simulink model "mass_spring_damper"  (R2026a)
settings: Solver=VariableStepAuto  StopTime=10

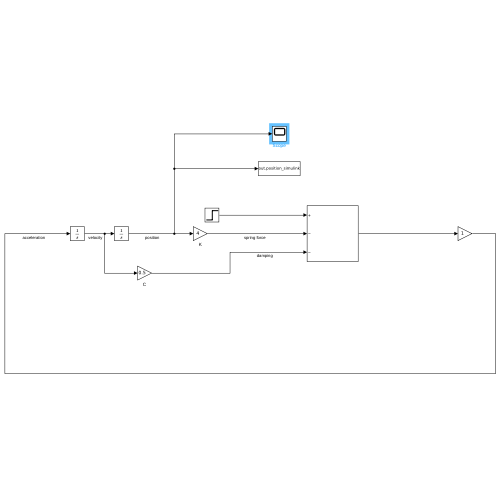
[thumbnail: Simulink's stored preview of the top-level diagram]
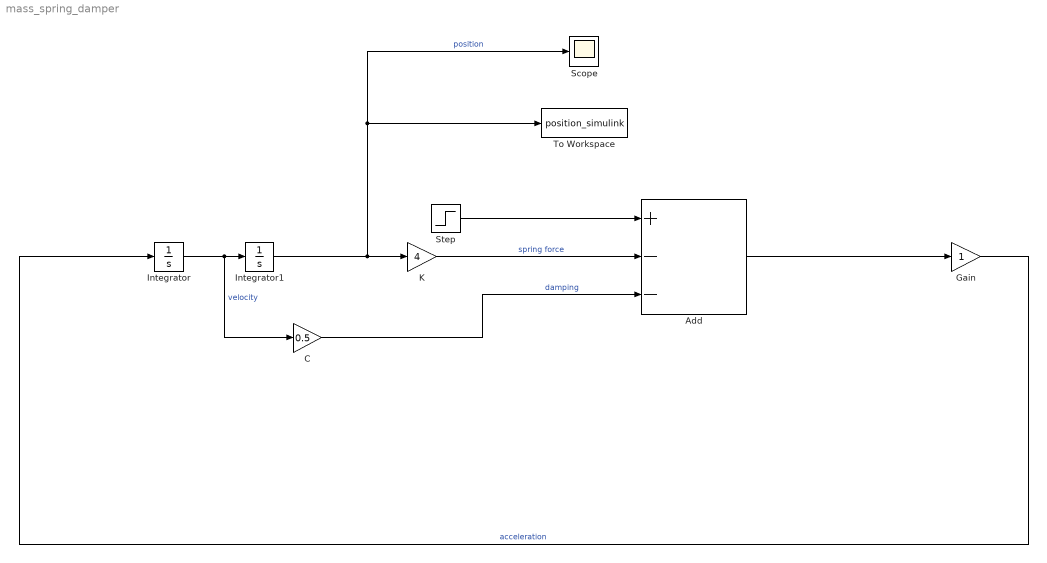
== system mass_spring_damper ==
  Add : Sum  Inputs=+--
  C : Gain  Gain=0.5
  Gain : Gain
  Integrator : Integrator
  Integrator1 : Integrator
  K : Gain  Gain=4
  Scope : Scope
      settings: ActiveDisplayYMinimum=-0.17646107003330896  ActiveDisplayYMaximum=0.553347101046636
  Step : Step  Time=0  SampleTime=0
  To Workspace : ToWorkspace  VariableName=position_simulink  SaveFormat=Timeseries  SampleTime=-1
  wires:
  Step/1 -> Add/1
  Gain/1 -> Integrator/1  "acceleration"
  Integrator/1 -> C/1, Integrator1/1  "velocity"
  Integrator1/1 -> To Workspace/1, Scope/1, K/1  "position"
  C/1 -> Add/3  "damping"
  K/1 -> Add/2  "spring force"
  Add/1 -> Gain/1
